simulink library "calc_path_length"  (R2022a)
settings: Solver=VariableStepAuto  StartTime=0.0  StopTime=10.0  RelTol=1e-3
settings Model: Creator=Ayaz  LastModifiedBy=lhill8
settings SolverCC: AlgebraicLoopSolver=TrustRegion
settings DebuggingCC: UnconnectedInputMsg=warning  UnconnectedOutputMsg=warning  UnconnectedLineMsg=warning  SFMachineParentedDataDiag=warning

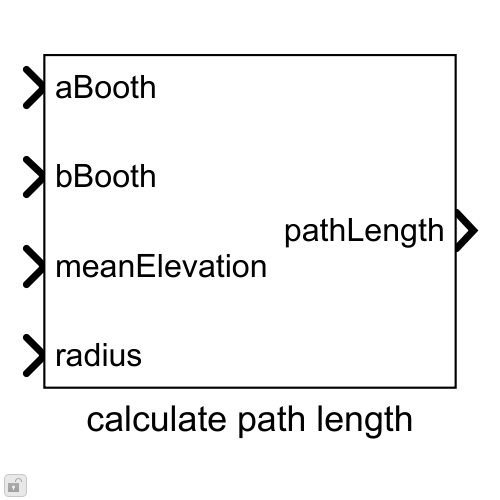
[thumbnail: Simulink's stored preview of the top-level diagram]
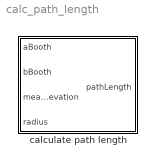
== system calc_path_length ==
  calculate path length : Subsystem

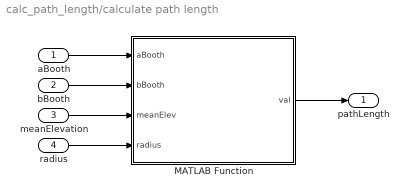
== system calc_path_length/calculate path length ==
  aBooth : Inport
  bBooth : Inport  Port=2
  meanElevation : Inport  Port=3
  radius : Inport  Port=4
  MATLAB Function : MATLAB Function  TreatAsAtomicUnit=on
  pathLength : Outport
  wires:
  aBooth/1 -> MATLAB Function/1(aBooth)
  bBooth/1 -> MATLAB Function/2(bBooth)
  meanElevation/1 -> MATLAB Function/3(meanElev)
  radius/1 -> MATLAB Function/4(radius)
  MATLAB Function/1(val) -> pathLength/1

== matlab function calc_path_length/calculate path length/MATLAB Function ==
  data: aBooth input; val output; bBooth input; meanElev input; radius input
function val = calcPathLength(aBooth,bBooth,meanElev,radius)

val = calcPathLength(aBooth,bBooth,meanElev,radius);

end
